simulink model "trans_2015a"  (R2015a)
settings: Solver=ode45  SolverMode=SingleTasking  StartTime=0.0  StopTime=10.0  RelTol=1e-3
InitFcn:
  | cd(tempdir)
  | clearvars
  | clc
  | 
  | %Carrossel?
  | mode_t=1;
  | 
  | %Parâmetros do transmissor
  | fs_Tx=200e3;
  | f_bits=10e3;
  | rolloff=0.5;
  | smpl_per_symb=5;
  | [N,D]=rat(400000/(f_bits*smpl_per_symb));
  | rate_inter=(N);
  | rate_dec=(D);
  | 
  | %data='The man in black fled across the desert, and the gunslinger followed. The desert was the apotheosis of all deserts, huge, standing to the sky for what might have been parsecs in all directions. White; blinding; waterless; without feature save for the faint, cloudy haze of the mountains which sketched themselves on the horizon and the devil-grass which brought sweet dreams, nightmares, death. An occasional tombstone sign pointed the way, for once the drifted track that cut its way through the thick crust of alkali had been a highway and coaches had followed it. The world had moved on since then. The world had emptied. The gunslinger walked stolidly, not hurrying, not loafing. A hide waterbag was slung around his middle like a bloated sausage. It was almost full. He had progressed through the khef over many years, and had reached the fifth level. At the seventh or eighth, he would not have been thirsty; he could have watched own body dehydrate with clinical, detached attention, watering its crevices and dark inner hollows only when his logic told him it must be done. He was not seventh or eighth. He was fifth. So he was thirsty, although he had no particular urge to drink. In a vague way, all this pleased him. It was romantic. Below the waterbag were his guns, finely weighted to his hand. The two belts crisscrossed above his crotch. The holsters were oiled too deeply for even this Philistine sun to crack. The stocks of the guns were sandalwood, yellow and finely grained. The holsters were tied down with raw hide cord, and they swung heavily against his hips. The brass casings of the cartridges looped into the gun belts twinkled and flashed and heliographed in the sun. The leather made subtle creaking noises. The guns themselves made no noise. They had spilled blood. There was no need to make noise in the sterility of the desert His clothes were the no-color of rain or dust. His shirt was open at the throat, with a rawhide thong dangling loosely in hand-punched eyelets. His pants were seam-stretched dungarees. He breasted a gently rising dune (although there was no sand here; the desert was hardpan, and even the harsh winds that blew when dark came raised only an aggravating harsh dust like scouring powder) and saw the kicked remains of a tiny campfire on the lee side, the side which the sun would quit earliest. Small signs like this, once more affirming the man in black´s essential humanity, never failed to please him. His lips stretched in the pitted, flaked remains of his face. He squatted. He had burned the devil-grass, of course. It was the only thing out here that would burn. It burned with a greasy, flat light, and it burned slow. Border dwellers had told him that devils lived even in the flames. They burned it but would not look into the light. They said the devils hypnotized, beckoned, would eventually draw the one who looked into the fires. And the next man foolish enough to look into the fire might see you. The burned grass was crisscrossed in the now-familiar ideographic pattern, and crumbled to gray senselessness before the gunslinger´s prodding hand. There was nothing in the remains but a charred scrap of bacon, which he ate thoughtfully. It had always been this way. The gunslinger had followed the man in black across the desert for two months now, across the endless, screamingly monotonous purgatorial wastes, and had yet to find spoor other than the hygienic sterile ideographs of the man in black´s camp fires. He had not found a can, a bottle, or a waterbag (the gunslinger had left four of those behind, like dead snake-skins).';
  | data='The man in black fled across the desert, and the gunslinger followed. The desert was the apotheosis of all deserts, huge, standing to the sky for what might have been parsecs in all directions. White; blinding; waterless; without feature save for the faint, cloudy haze of the mountains which sketched themselves on the horizon and the devil-grass which brought sweet dreams, nightmares, death. An occasional tombstone sign pointed the way, for once the drifted track that cut its way through the thick crust of alkali had been a highway and coaches had followed it. The world had moved on since then.';
undefined symbols (not defined in the file): firnyquist
libraries: rtlsdr_book_library x1, dspmlti4 x1, commdigbbndpm3 x1, commfilt2 x1
settings Model: CovMetricSettings=dwe  CovHtmlReporting=off  covSaveCumulativeToWorkspaceVar=off  CovSaveSingleToWorkspaceVar=off  CovExternalEMLEnable=on  Creator=Enrique Pinto  LastModifiedBy=Enrique Pinto
settings DataIOCC: LimitDataPoints=off  SaveFormat=Dataset
settings DebuggingCC: SFUnexpectedBacktrackingDiag=error  SFNoUnconditionalDefaultTransitionDiag=error
settings HardwareCC: ProdBitPerPointer=64  ProdLargestAtomicFloat=Float  ProdIntDivRoundTo=Zero  ProdEndianess=LittleEndian  ProdHWDeviceType=Specified
settings ModelReferenceCC: PropagateSignalLabelsOutOfModel=on
settings GRTTargetCC: TargetLangStandard=C99 (ISO)  GeneratePreprocessorConditionals=Use local settings

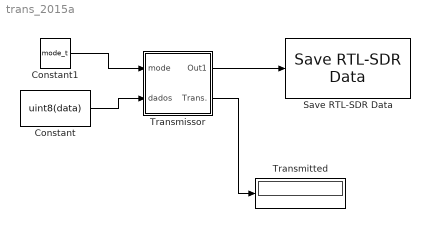
== system trans_2015a ==
  Constant : Constant  Value=uint8(data)
  Constant1 : Constant  Value=mode_t
  Save RTL-SDR Data : rtlsdr_book_library/Additional Tools/Save RTL-SDR Data  file_name=C:\Users\Enrique Pinto\Desktop\SDR\Projeto\trans_data.mat
  Transmissor : Subsystem
  Transmitted : Display
  wires:
  Constant/1 -> Transmissor/2(dados)
  Constant1/1 -> Transmissor/1(mode)
  Transmissor/2(Trans.) -> Transmitted/1
  Transmissor/1(Out1) -> Save RTL-SDR Data/1

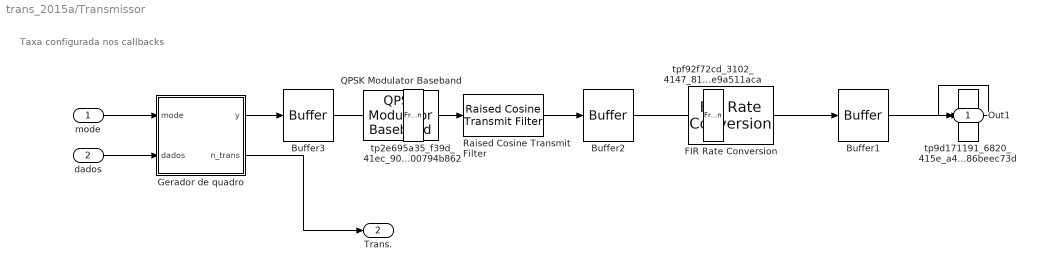
== system trans_2015a/Transmissor ==
  note: Taxa configurada nos callbacks
  mode : Inport
  dados : Inport  Port=2
  Buffer1 : Buffer  N=1000
  Buffer2 : Buffer  N=1000
  Buffer3 : Buffer  N=2
  FIR Rate Conversion : dspmlti4/FIR Rate Conversion  FilterSource=Specify via dialog  L=rate_inter  h=rate_inter .* firnyquist(24*max(rate_inter,rate_dec), max(rate_inter,rate_dec), kaiser(1 + 24*max(rate_inter,rate_dec), 0.1102*(80-8.71)))  M=rate_dec  FilterObject=FRC  roundingMode=Floor  overflowMode=off  firstCoeffDataTypeStr=Inherit: Same word length as input  firstCoeffMin=[]  firstCoeffMax=[]  firstCoeffLastDataTypeStr=Inherit: Same word length as input  outputDataTypeStr=Inherit: Same as accumulator  outputMin=[]  outputMax=[]  outputLastDataTypeStr=Inherit: Same as accumulator
  Gerador de quadro : MATLAB Function  TreatAsAtomicUnit=on  SystemSampleTime=1000/(f_bits)
      settings: PermitHierarchicalResolution=ParametersOnly
  QPSK Modulator Baseband : commdigbbndpm3/QPSK Modulator Baseband  InType=Bit  Enc=Gray  Ph=pi/4  outDtype=double  outWordLen=16  outUDDataType=sfix(16)  outFracLenMode=Best precision  outFracLen=15
  Raised Cosine Transmit Filter : commfilt2/Raised Cosine Transmit Filter  filtType=Square root  R=rolloff  filtSpan=10  N=smpl_per_symb  filterGain=1  InputProcessing=Columns as channels (frame based)  framing=Enforce single-rate processing  checkCoeff=off  variableName=rcTxFilt  checkGain=Normalized  sampMode=Mute  saveAsFlag=1  currentFiltSpan=10  D=(10)/2  launchFVT=on  roundingMode=Floor  overflowMode=off
  tp2e695a35_f39d_41ec_9008_c3500794b862 : FrameConversion  InheritSamplingMode=off  OutFrame=Sample-based
  tp9d171191_6820_415e_a4ee_bf786beec73d : FrameConversion  InheritSamplingMode=off  OutFrame=Sample-based
  tpf92f72cd_3102_4147_81a1_ab8e9a511aca : FrameConversion  InheritSamplingMode=off  OutFrame=Sample-based
  Out1 : Outport
  Trans. : Outport  Port=2
  wires:
  FIR Rate Conversion/1 -> Buffer1/1
  Gerador de quadro/1(y) -> Buffer3/1
  mode/1 -> Gerador de quadro/1(mode)
  dados/1 -> Gerador de quadro/2(dados)
  QPSK Modulator Baseband/1 -> Raised Cosine Transmit Filter/1
  Gerador de quadro/2(n_trans) -> Trans./1
  Raised Cosine Transmit Filter/1 -> Buffer2/1
  Buffer1/1 -> tp9d171191_6820_415e_a4ee_bf786beec73d/1
  tp9d171191_6820_415e_a4ee_bf786beec73d/1 -> Out1/1
  Buffer2/1 -> tpf92f72cd_3102_4147_81a1_ab8e9a511aca/1
  tpf92f72cd_3102_4147_81a1_ab8e9a511aca/1 -> FIR Rate Conversion/1
  Buffer3/1 -> tp2e695a35_f39d_41ec_9008_c3500794b862/1
  tp2e695a35_f39d_41ec_9008_c3500794b862/1 -> QPSK Modulator Baseband/1

== matlab function trans_2015a/Transmissor/Gerador de quadro ==
  data: mode input; y output; dados input; n_trans output
function [y,n_trans] = fcn(mode,dados)
persistent databuf;
if isempty(databuf)
    %A opção abaixo funciona
    %databuf=uint8('The man in black fled across the desert, and the gunslinger followed. The desert was the apotheosis of all deserts, huge, standing to the sky for what might have been parsecs in all directions. White; blinding; waterless; without feature save for the faint, cloudy haze of the mountains which sketched themselves on the horizon and the devil-grass which brought sweet dreams, nightmares, death. An occasional tombstone sign pointed the way, for once the drifted track that cut its way through the thick crust of alkali had been a highway and coaches had followed it. The world had moved on since then. The world had emptied. The gunslinger walked stolidly, not hurrying, not loafing. A hide waterbag was slung around his middle like a bloated sausage. It was almost full. He had progressed through the khef over many years, and had reached the fifth level. At the seventh or eighth, he would not have been thirsty; he could have watched own body dehydrate with clinical, detached attention, watering its crevices and dark inner hollows only when his logic told him it must be done. He was not seventh or eighth. He was fifth. So he was thirsty, although he had no particular urge to drink. In a vague way, all this pleased him. It was romantic. Below the waterbag were his guns, finely weighted to his hand. The two belts crisscrossed above his crotch. The holsters were oiled too deeply for even this Philistine sun to crack. The stocks of the guns were sandalwood, yellow and finely grained. The holsters were tied down with raw hide cord, and they swung heavily against his hips. The brass casings of the cartridges looped into the gun belts twinkled and flashed and heliographed in the sun. The leather made subtle creaking noises. The guns themselves made no noise. They had spilled blood. There was no need to make noise in the sterility of the desert His clothes were the no-color of rain or dust. His shirt was open at the throat, with a rawhide thong dangling loosely in hand-punched eyelets. His pants were seam-stretched dungarees. He breasted a gently rising dune (although there was no sand here; the desert was hardpan, and even the harsh winds that blew when dark came raised only an aggravating harsh dust like scouring powder) and saw the kicked remains of a tiny campfire on the lee side, the side which the sun would quit earliest. Small signs like this, once more affirming the man in black´s essential humanity, never failed to please him. His lips stretched in the pitted, flaked remains of his face. He squatted. He had burned the devil-grass, of course. It was the only thing out here that would burn. It burned with a greasy, flat light, and it burned slow. Border dwellers had told him that devils lived even in the flames. They burned it but would not look into the light. They said the devils hypnotized, beckoned, would eventually draw the one who looked into the fires. And the next man foolish enough to look into the fire might see you. The burned grass was crisscrossed in the now-familiar ideographic pattern, and crumbled to gray senselessness before the gunslinger´s prodding hand. There was nothing in the remains but a charred scrap of bacon, which he ate thoughtfully. It had always been this way. The gunslinger had followed the man in black across the desert for two months now, across the endless, screamingly monotonous purgatorial wastes, and had yet to find spoor other than the hygienic sterile ideographs of the man in black´s camp fires. He had not found a can, a bottle, or a waterbag (the gunslinger had left four of those behind, like dead snake-skins).$$$$$$$$$$$$$$$$$$$$$$$$$$$$$$$$');
    %A opção abaixo carrega no buffer apenas o primeiro elemento de dados!
    databuf=uint8(zeros(1,length(dados)));
    databuf(1:length(dados))=dados(1:length(dados));
end
persistent i;
if isempty(i)
    i=1;
end
persistent n_count;
if isempty(n_count)
    n_count=0;
end
frame=zeros(1,984);
%Barker 13 =>[1 1 1 1 1 0 0 1 1 0 1 0 1]
%Preâmbulo de sincronismo
frame(1:52)=[1 1 1 1 1 1 1 1 1 1 0 0 0 0 1 1 1 1 0 0 1 1 0 0 1 1 1 1 1 1 1 0 0 1 1 0 1 0 1 1 1 1 1 1 0 0 1 1 0 1 0 1];
%Modo
frame(53:55)=zeros(1,3);
frame(56)=mode;

%Índice
frame(57:64-size(de2bi(i-1),2))=zeros(1,8-size(de2bi(i-1),2));
frame(64-size(de2bi(i-1),2)+1:64)=fliplr(de2bi(i-1));

%End_flag e carrossel
texto=uint8('vazio');
texto=texto';

databuf=uint8(zeros(1,length(dados)));
databuf(1:length(dados))=dados(1:length(dados));
    
if(mode==1)%verifica se é carrossel
    carrossel_size=ceil(size(databuf,2)/114);
    if(i==carrossel_size)
        frame(65)=1;
        texto=databuf((i-1)*114+1:(size(databuf,2)));
        i=1;
    else
        if(i<carrossel_size)
            texto=databuf((i-1)*114+1:i*114);
            i=i+1;
        else
            i=1;
        end
    end
else
    texto=databuf(1:114);
    texto=texto.';
    if(i==256)
        frame(65)=1;
        i=1;
    else
        if(i<256)
            i=i+1;
        else
            i=1;
        end
    end
end

%Tamanho mensagem
frame(66:72-size(dec2bin(size(dec2bin(texto),1)),2))=zeros(1,7-size(dec2bin(size(dec2bin(texto),1)),2));
frame(72-size(dec2bin(size(dec2bin(texto),1)),2)+1:72)=dec2bin(size(dec2bin(texto),1));
%Dados
mensagem = reshape(dec2bin(texto, 8).'-'0',1,[]);
frame(73:73+size(mensagem,2)-1)=mensagem';
frame(73+size(mensagem,2):984)=randi([0 1],1,984-(73+size(mensagem,2))+1);
%Output
H = comm.CRCGenerator;
y_sem_pre=step(H,frame(53:end)');
y=[frame(1:52)'; y_sem_pre];
n_count=n_count+1;
n_trans=n_count;
